simulink model "id_model"  (R2019b)
settings: Solver=VariableStepAuto  StartTime=0.0  StopTime=10.0  RelTol=1e-3
undefined symbols (not defined in the file or in its folder): DEN, DENr, NUM, NUMr
settings Model: Creator=Merc  LastModifiedBy=brian
settings DataIOCC: ReturnWorkspaceOutputs=off
settings DebuggingCC: ArithmeticOperatorsInVariantConditions=warning
settings SFSimCC: CustomCodeUndefinedFunction=UseInterfaceOnly

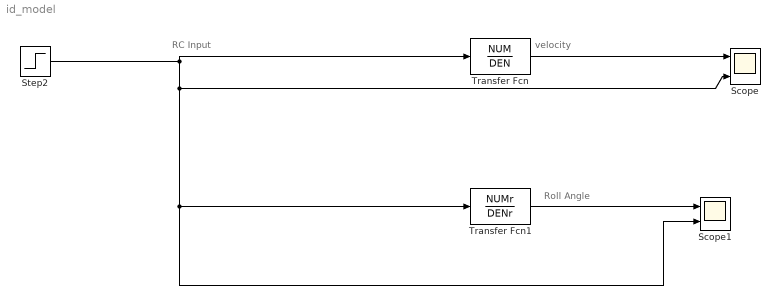
== system id_model ==
  note: Roll Angle
  note: RC Input
  note: velocity
  Scope : Scope  NumInputPorts=2
  Scope1 : Scope  NumInputPorts=2
  Step2 : Step  Time=2  After=100  SampleTime=0
  Transfer Fcn : TransferFcn  Numerator=NUM  Denominator=DEN
  Transfer Fcn1 : TransferFcn  Numerator=NUMr  Denominator=DENr
  wires:
  Step2/1 -> Scope/2, Transfer Fcn1/1, Scope1/2, Transfer Fcn/1
  Transfer Fcn1/1 -> Scope1/1
  Transfer Fcn/1 -> Scope/1
